simulink model "water_hopper_cpg"  (Simulink 8.0)
settings: Solver=ode23t  StartTime=0.0  StopTime=5  MaxStep=1e-3  RelTol=1e-9
values from neighbouring files (symbols this model uses):
  alpha = 30    [SimParam.m]    (also in SimParam_cpg.m)
  Amp = coeff(1)    [SSheight3.m]    (also in SimParam.m = 0.0249; SimParam_cpg.m = 0.0249; TwoD_search.m = AMP(jj,1); linear_search.m = leg_length/4)
  amp = Amp    (= 0.0249)    [SimParam.m]    (also in SimParam_cpg.m)
  b = 0.5*C_d*S*density    [SSheight.m]    (also in SSheight12.m; SSheight2.m; SSheight3.m; SSpower.m)
  C_d = 0.703    [SSheight.m]    (also in SSheight12.m; SSheight2.m; SSheight3.m; SSpower.m)
  density = 1000    [SSheight.m]    (also in SSheight12.m; SSheight2.m; SSheight3.m; SSpower.m)
  Fratio = (r2^2)/(r1^2)    (= 0.0625)    [SimParam_cpg.m]
  freq = 84    [SimParam_cpg.m]    (also in TwoD_search.m = FREQ(1,kk); height_search.m = FREQ(k); height_search2.m = freqs(k); linear_search.m = FREQ(2:end))
  g = 9.81    [SSheight.m]    (also in SSheight12.m; SSheight2.m; SSheight3.m; SSpower.m)
  k = C_d*S*density*g    [SSheight.m]    (also in SSheight12.m; SSheight2.m; SSheight3.m; SSpower.m)
  leg_length = Amp    (= 0.0249)    [SimParam.m]    (also in SimParam_2G.m = 0.1; SimParam_cpg.m; height_search.m = Amp)
  mass = 0.025    [SimParam.m]    (also in SimParam_cpg.m)
  omega_0 = [65 65]'    [SimParam_cpg.m]
  S1 = (pi*r1^2)*area    (= 0.00115422114093)    [SimParam.m]    (also in SimParam_cpg.m)
  S2 = (pi*r2^2)*area    (= 7.21388213081e-05)    [SimParam.m]    (also in SimParam_cpg.m)
  tau = 0.001    [SimParam.m]    (also in SimParam_cpg.m)
  y_0 = Amp/2    (= 0.01245)    [SimParam.m]    (also in SimParam_2G.m = 0.1; SimParam_cpg.m; height_search.m = Amp/2; height_search2.m = Amp/2)
libraries: mblibv1 x13, simulink x2, dspinverses x1, powerlib_extras x1
settings Model: Creator=Metti  LastModifiedBy=nitisht
settings SolverCC: ZeroCrossControl=DisableAll
settings DataIOCC: SignalLoggingSaveFormat=ModelDataLogs
settings DebuggingCC: FcnCallInpInsideContextMsg=EnableAllAsWarning
settings SimMechanicsCC: VisSampleTime=0.05  AutoFitVis=GROWTOFIT  LastVizWinPosition=[520 378 560 420]  CamPosition=[0;32.5432;11.11;]  CamTarget=[0;32.5432;0;]  CamUpVector=[0;1;0;]  CamHeight=0.102  VisBackgroundColor=[0.9;0.9;0.95;]  DefaultBodyColor=[1;0;0;]
settings ConfigurationSet: Description=SimMechanics 2G

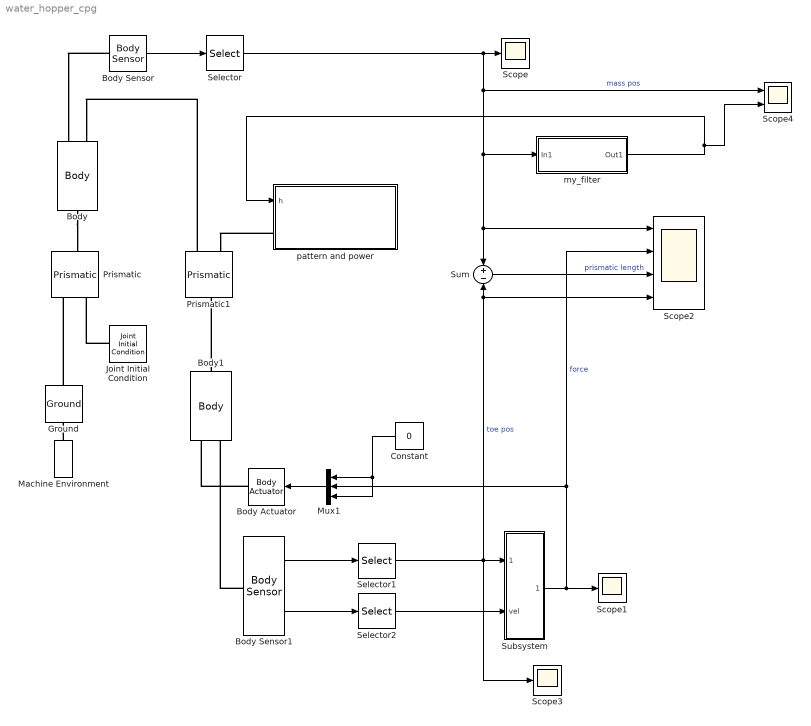
== system water_hopper_cpg ==
  Body : mblibv1/Bodies/Body  LConnTagsString=CS1  RConnTagsString=CS2|CS3  UpdateFromCAD=off  DialogClass=MechanicalBodyBlock  Mass=mass  MassUnits=kg  InertiaUnits=kg*m^2  Inertia=eye(3)  Shape=Cylinder  ShapeDims=[1 1]  ShapeUnits=m  ShapeUse=false  Density=1  DensityUnits=kg/m^3  DensityUse=false  GraphicsMode=MACHINE_DEFAULT  BodyColorSelMode=MACHINE_DEFAULT  BodyColor=[1 0 0]  AttachedToCS=CG  CG=Left$CG$[0 0 0]$WORLD$WORLD$m$[0 0 0]$Euler X-Y-Z$deg$WORLD$false$none  WorkingFrames=Left$CS1$[0 0 0]$CG$CG$m$[0 0 0]$Euler X-Y-Z$deg$WORLD$true$none#Right$CS2$[0 0 0]$CG$CG$m$[0 0 0]$Euler X-Y-Z$deg$WORLD$true$none#Right$CS3$[0 0 0]$CG$CG$m$[0 0 0]$Euler X-Y-Z$deg$WORLD$true$none  CGPos=[0 0 0]  CGRot=[0 0 0]  CS0Pos=[]  CS0Rot=[]  CS1Pos=[0 0 0]  CS1Rot=[0 0 0]  CS2Pos=[0 0 0]  CS2Rot=[0 0 0]  CS3Pos=[0 0 0]  CS3Rot=[0 0 0]  CS4Pos=[]  CS4Rot=[]  CS5Pos=[]  CS5Rot=[]  CS6Pos=[]  CS6Rot=[]  CS7Pos=[]  CS7Rot=[]  CS8Pos=[]  CS8Rot=[]  CS9Pos=[]  CS9Rot=[]  CS10Pos=[]  CS10Rot=[]  CS11Pos=[]  CS11Rot=[]  CS12Pos=[]  CS12Rot=[]  CS13Pos=[]  CS13Rot=[]  CS14Pos=[]  CS14Rot=[]  CS15Pos=[]  CS15Rot=[]  CS16Pos=[]  CS16Rot=[]  CS17Pos=[]  CS17Rot=[]  CS18Pos=[]  CS18Rot=[]  CS19Pos=[]  CS19Rot=[]  CS20Pos=[]  CS20Rot=[]
  Body Actuator : mblibv1/Sensors &  Actuators/Body Actuator  UpdateFromCAD=off  PhysicalDomain=Mechanical  PortType=blob  ActuationStyle=Force  AngleUnits=deg  ArcVelocityUnits=deg/s  ArcAccelerationUnits=deg/s^2  CoordPositionUnits=m  VelocityUnits=m/s  AccelerationUnits=m/s^2  ForceUnits=N  TorqueUnits=N-m  ActiveIO=on  Width=3  DialogClass=MechanicalActuatorBlock  ReferenceFrame=Absolute (World)  Angle=off  CoordPosition=on  Force=on  Torque=off
  Body Sensor : mblibv1/Sensors &  Actuators/Body Sensor  UpdateFromCAD=off  PhysicalDomain=Mechanical  PortType=blob  Muxed=on  Pose=off  Angle=on  AngleUnits=deg  ArcVelocity=off  ArcVelocityUnits=deg/s  ArcAcceleration=off  ArcAccelerationUnits=deg/s^2  CoordPosition=on  CoordPositionUnits=m  Velocity=off  VelocityUnits=m/s  Acceleration=off  AccelerationUnits=m/s^2  Quaternion=on  QuaternionDT=off  QuaternionDDT=off  QuaternionUnits=off  OutputVector=[1]  ActiveIO=on  Width=3  DialogClass=MechanicalSensorBlock  ReferenceFrame=Absolute (World)
  Body Sensor1 : mblibv1/Sensors &  Actuators/Body Sensor  UpdateFromCAD=off  PhysicalDomain=Mechanical  PortType=blob  Muxed=off  Pose=off  Angle=on  AngleUnits=deg  ArcVelocity=off  ArcVelocityUnits=deg/s  ArcAcceleration=off  ArcAccelerationUnits=deg/s^2  CoordPosition=on  CoordPositionUnits=m  Velocity=on  VelocityUnits=m/s  Acceleration=off  AccelerationUnits=m/s^2  Quaternion=on  QuaternionDT=off  QuaternionDDT=off  QuaternionUnits=off  OutputVector=[1]  ActiveIO=on  Width=6  DialogClass=MechanicalSensorBlock  ReferenceFrame=Absolute (World)
  Body1 : mblibv1/Bodies/Body  LConnTagsString=CS1  RConnTagsString=CS2|CS3  UpdateFromCAD=off  DialogClass=MechanicalBodyBlock  Mass=0  MassUnits=kg  InertiaUnits=kg*m^2  Inertia=eye(3)  Shape=Cylinder  ShapeDims=[1 1]  ShapeUnits=m  ShapeUse=false  Density=1  DensityUnits=kg/m^3  DensityUse=false  GraphicsMode=MACHINE_DEFAULT  BodyColorSelMode=MACHINE_DEFAULT  BodyColor=[1 0 0]  AttachedToCS=CG  CG=Left$CG$[0 -leg_length 0]$CS1$CS1$m$[0 0 0]$Euler X-Y-Z$deg$WORLD$false$none  WorkingFrames=Left$CS1$[0 0 0]$Adjoining$Adjoining$m$[0 0 0]$Euler X-Y-Z$deg$WORLD$true$none#Right$CS2$[0 -leg_length 0]$CS1$CS1$m$[0 0 0]$Euler X-Y-Z$deg$WORLD$true$none#Right$CS3$[0 -leg_length 0]$CS1$CS1$m$[0 0 0]$Euler X-Y-Z$deg$WORLD$true$none  CGPos=[0 -leg_length 0]  CGRot=[0 0 0]  CS0Pos=[]  CS0Rot=[]  CS1Pos=[0 0 0]  CS1Rot=[0 0 0]  CS2Pos=[0 -leg_length 0]  CS2Rot=[0 0 0]  CS3Pos=[0 -leg_length 0]  CS3Rot=[0 0 0]  CS4Pos=[]  CS4Rot=[]  CS5Pos=[]  CS5Rot=[]  CS6Pos=[]  CS6Rot=[]  CS7Pos=[]  CS7Rot=[]  CS8Pos=[]  CS8Rot=[]  CS9Pos=[]  CS9Rot=[]  CS10Pos=[]  CS10Rot=[]  CS11Pos=[]  CS11Rot=[]  CS12Pos=[]  CS12Rot=[]  CS13Pos=[]  CS13Rot=[]  CS14Pos=[]  CS14Rot=[]  CS15Pos=[]  CS15Rot=[]  CS16Pos=[]  CS16Rot=[]  CS17Pos=[]  CS17Rot=[]  CS18Pos=[]  CS18Rot=[]  CS19Pos=[]  CS19Rot=[]  CS20Pos=[]  CS20Rot=[]
  Constant : Constant  Value=0
  Ground : mblibv1/Bodies/Ground  UpdateFromCAD=off  LeftPortType=env  RightPortType=workingframe  PhysicalDomain=Mechanical  DialogClass=GroundBlock  CoordPosition=[0 0 0]  CoordPositionUnits=m  StateVectorMgrId=1  MachineId=[2 0]  ShowEnvPort=on
  Joint Initial Condition : mblibv1/Sensors &  Actuators/Joint Initial Condition  UpdateFromCAD=off  LeftPortType=blob  RightPortType=blob  PhysicalDomain=mechanical  DialogClass=InitialConditionBlock  InitialConditions=P1$true$y_0$m$deg$0$m/s$deg/s#P2$false$0$m$deg$0$m/s$deg/s#P3$false$0$m$deg$0$m/s$deg/s#R1$false$0$m$deg$0$m/s$deg/s#R2$false$0$m$deg$0$m/s$deg/s#R3$false$0$m$deg$0$m/s$deg/s#S$false$0$m$deg$0$m/s$deg/s  P1PIC=y_0  P1VIC=0  P2PIC=0  P2VIC=0  P3PIC=0  P3VIC=0  R1PIC=0  R1VIC=0  R2PIC=0  R2VIC=0  R3PIC=0  R3VIC=0  SPIC=0  SVIC=0
  Machine Environment : mblibv1/Bodies/Machine Environment  PortType=env  PhysicalDomain=Mechanical  DialogTemplateClass=MECH.MachineEnvironment  SyncWhenCopied=off  Gravity=[0 -g 0]  GravityUnits=m/s^2  GravityAsSignal=off  Dimensionality=Auto-detect  AnalysisType=Forward dynamics  LinearAssemblyTolerance=1e-3  LinearAssemblyToleranceUnits=m  AngularAssemblyTolerance=1e-3  AngularAssemblyToleranceUnits=rad  ConstraintSolverType=Stabilizing  ConstraintRelTolerance=1e-4  ConstraintAbsTolerance=1e-4  UseRobustSingularityHandling=off  RedundancyAnalysisToleranceType=Automatically select tolerance  RedundancyAnalysisTolerance=1e-14  StatePerturbationType=Fixed  PerturbationSize=1e-5  VisualizeMachine=on  BodyVisualizationType=Use model default body geometries  BodyColorSelMode=Use model default  DefaultBodyColor=[1 0 0]
  Mux1 : Mux  Inputs=3
  Prismatic : mblibv1/Joints/Prismatic  LConnTagsString=__newl0|SA1  RConnTagsString=__newr0  UpdateFromCAD=off  NumSAPorts=1  CutJoint=off  MarkAsCut=off  Primitives=prismatic  PrimitiveProps=P1$World$[0 1 0]$prismatic  DialogClass=JointBlock  P1Axis=[0 1 0]
  Prismatic1 : mblibv1/Joints/Prismatic  LConnTagsString=__newl0|SA1  RConnTagsString=__newr0  UpdateFromCAD=off  NumSAPorts=1  CutJoint=off  MarkAsCut=off  Primitives=prismatic  PrimitiveProps=P1$World$[0 1 0]$prismatic  DialogClass=JointBlock  P1Axis=[0 1 0]
  Scope : Scope
      settings: YMin=-0.053045  YMax=-0.053005  SaveName=ball_position
  Scope1 : Scope
      settings: SaveName=force
  Scope2 : Scope  NumInputPorts=4
      settings: YMin=-5~-5~-5~-5  YMax=5~5~5~5  SaveName=ScopeData2
  Scope3 : Scope
      settings: SaveName=toe_position
  Scope4 : Scope  NumInputPorts=2
      settings: YMin=-0.015~0.009  YMax=0.03~0.02  SaveName=ball_position1
  Selector : Selector  InputPortWidth=3  IndexOptions=Index vector (dialog)  Indices=[2]  OutputSizes=1
  Selector1 : Selector  InputPortWidth=3  IndexOptions=Index vector (dialog)  Indices=[2]  OutputSizes=1
  Selector2 : Selector  InputPortWidth=3  IndexOptions=Index vector (dialog)  Indices=[2]  OutputSizes=1
  Subsystem : Subsystem
  Sum : Sum  Inputs=+|-
  my_filter : Subsystem
  pattern and power : Subsystem
  wires:
  Body Sensor/1 -> Selector/1
  Selector/1 -> Scope/1, Scope4/1, Scope2/1, Sum/1, my_filter/1(In1)  "mass pos"
  Body Sensor1/1 -> Selector1/1
  Body Sensor1/2 -> Selector2/1
  Selector1/1 -> Sum/2, Scope2/4, Subsystem/1(pos), Scope3/1  "toe pos"
  Selector2/1 -> Subsystem/2(vel)
  Subsystem/1(force) -> Scope1/1, Mux1/2, Scope2/2  "force"
  Mux1/1 -> Body Actuator/1
  Constant/1 -> Mux1/1, Mux1/3
  Sum/1 -> Scope2/3  "prismatic length"
  my_filter/1(Out1) -> pattern and power/1(h), Scope4/2
  connections:
  Body Sensor/LConn1 -- Body/RConn1
  Body/LConn1 -- Prismatic/RConn1
  Machine Environment/RConn1 -- Ground/LConn1
  Ground/RConn1 -- Prismatic/LConn1
  Body1/LConn1 -- Prismatic1/RConn1
  Body Actuator/RConn1 -- Body1/RConn1
  Body Sensor1/LConn1 -- Body1/RConn2
  Prismatic1/LConn1 -- Body/RConn2
  Joint Initial Condition/RConn1 -- Prismatic/LConn2
  pattern and power/LConn1 -- Prismatic1/LConn2

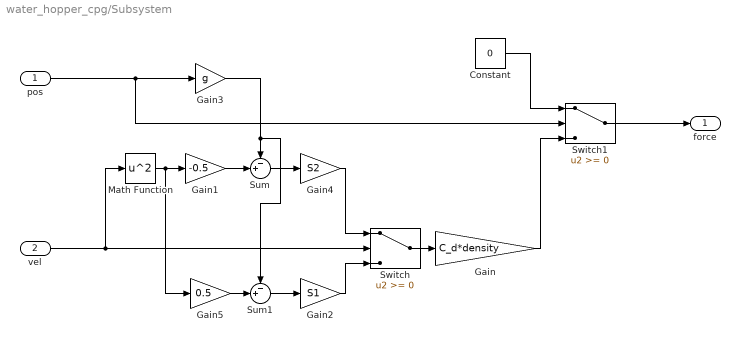
== system water_hopper_cpg/Subsystem ==
  pos : Inport
  vel : Inport  Port=2
  Constant : Constant  Value=0
  Gain : Gain  Gain=C_d*density
  Gain1 : Gain  Gain=-0.5
  Gain2 : Gain  Gain=S1
  Gain3 : Gain  Gain=g
  Gain4 : Gain  Gain=S2
  Gain5 : Gain  Gain=0.5
  Math Function : Math  Operator=square  SaturateOnIntegerOverflow=on
  Sum : Sum  Inputs=-+|
  Sum1 : Sum  Inputs=-+|
  Switch : Switch  ZeroCross=off
  Switch1 : Switch
  force : Outport
  wires:
  vel/1 -> Switch/2, Math Function/1
  Math Function/1 -> Gain1/1, Gain5/1
  Gain1/1 -> Sum/2
  pos/1 -> Gain3/1, Switch1/2
  Gain3/1 -> Sum/1, Sum1/1
  Sum/1 -> Gain4/1
  Gain4/1 -> Switch/1
  Gain2/1 -> Switch/3
  Switch/1 -> Gain/1
  Switch1/1 -> force/1
  Gain/1 -> Switch1/3
  Constant/1 -> Switch1/1
  Sum1/1 -> Gain2/1
  Gain5/1 -> Sum1/2

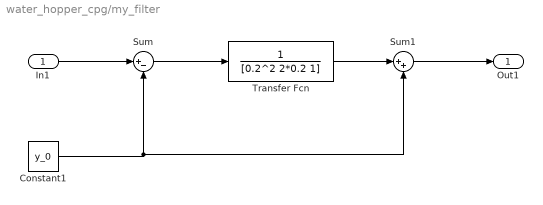
== system water_hopper_cpg/my_filter ==
  In1 : Inport
  Constant1 : Constant  Value=y_0
  Sum : Sum  Inputs=|+-
  Sum1 : Sum  Inputs=|++
  Transfer Fcn : TransferFcn  Denominator=[0.2^2 2*0.2 1]
  Out1 : Outport
  wires:
  Constant1/1 -> Sum1/2, Sum/2
  In1/1 -> Sum/1
  Sum/1 -> Transfer Fcn/1
  Transfer Fcn/1 -> Sum1/1
  Sum1/1 -> Out1/1

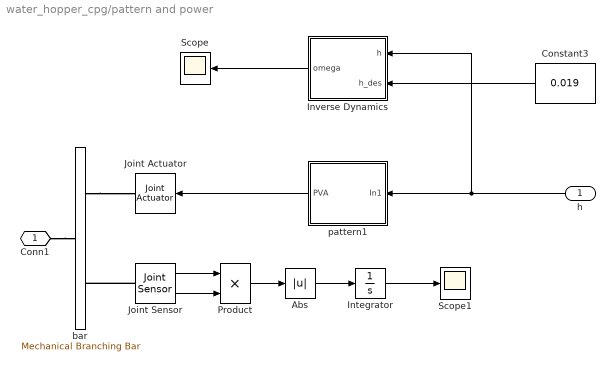
== system water_hopper_cpg/pattern and power ==
  h : Inport
  Abs : Abs
  Constant3 : Constant  Value=0.019
  Integrator : Integrator
  Inverse Dynamics : Subsystem
  Joint Actuator : mblibv1/Sensors &  Actuators/Joint Actuator  UpdateFromCAD=off  PhysicalDomain=Mechanical  PortType=blob  ActuationStyle=Motion  AngleUnits=deg  ArcVelocityUnits=deg/s  ArcAccelerationUnits=deg/s^2  CoordPositionUnits=m  VelocityUnits=m/s  AccelerationUnits=m/s^2  ForceUnits=N  TorqueUnits=N*m  ActiveIO=on  Width=3  DialogClass=MechanicalActuatorBlock  Primitive=P1  ReferenceFrame=Absolute (World)
  Joint Sensor : mblibv1/Sensors &  Actuators/Joint Sensor  UpdateFromCAD=off  PhysicalDomain=Mechanical  PortType=blob  Muxed=off  Pose=off  Angle=on  AngleUnits=deg  ArcVelocity=off  ArcVelocityUnits=deg/s  ArcAcceleration=off  ArcAccelerationUnits=deg/s^2  CoordPosition=off  CoordPositionUnits=m  Velocity=on  VelocityUnits=m/s  Acceleration=off  AccelerationUnits=m/s^2  Quaternion=on  QuaternionDT=off  QuaternionDDT=off  QuaternionUnits=off  OutputVector=[1]  ActiveIO=on  Width=2  DialogClass=MechanicalSensorBlock  Primitive=P1  Force=on  ForceUnits=N  Torque=off  TorqueUnits=N*m  ReferenceFrame=Absolute (World)  ReactionSensedSide=Base  ReactionReferenceFrame=Absolute (World)  ReactionForce=off  ReactionForceUnits=N  ReactionMoment=off  ReactionMomentUnits=N*m
  Product : Product  RndMeth=Zero
  Scope : Scope
      settings: YMin=62.5  YMax=90  SaveName=ScopeData5
  Scope1 : Scope
      settings: SaveName=Work
  bar : mblibv1/Utilities/Mechanical Branching Bar  LConnTagsString=_newl0  RConnTagsString=SA0|SA1  UpdateFromCAD=off  DialogClass=MechanicalBranchingBarBlock  NumSAPorts=2
  pattern1 : Subsystem  mask{Amp=amp, Offset=0, freq=freq}
      mask prompts: Amp "Amplitude"; freq "Frequency"
      mask TypeOptions freq: Constant/Value
  Conn1 : PMIOPort  Port=1  Side=Left
  wires:
  pattern1/1(PVA) -> Joint Actuator/1
  Joint Sensor/1 -> Product/1
  Product/1 -> Abs/1
  Abs/1 -> Integrator/1
  Integrator/1 -> Scope1/1
  Joint Sensor/2 -> Product/2
  h/1 -> Inverse Dynamics/1(h), pattern1/1(In1)
  Constant3/1 -> Inverse Dynamics/2(h_des)
  Inverse Dynamics/1(omega) -> Scope/1
  connections:
  bar/RConn1 -- Joint Actuator/RConn1
  Joint Sensor/LConn1 -- bar/RConn2
  Conn1/RConn1 -- bar/LConn1

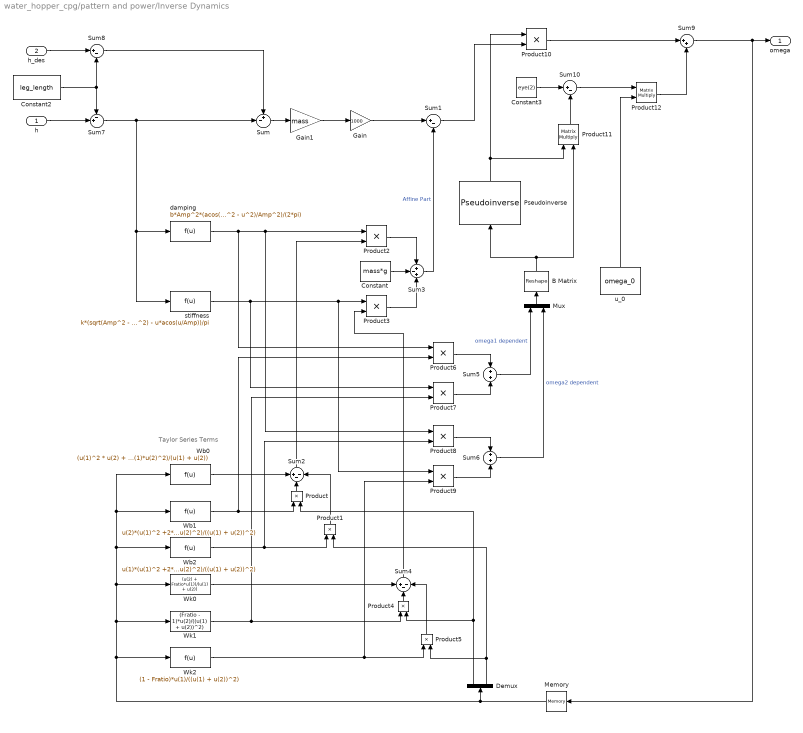
== system water_hopper_cpg/pattern and power/Inverse Dynamics ==
  note: Taylor Series Terms
  h : Inport
  h_des : Inport  Port=2
  B Matrix : Reshape  OutputDimensionality=Customize  OutputDimensions=[1,2]
  Constant : Constant  Value=mass*g
  Constant2 : Constant  Value=leg_length
  Constant3 : Constant  Value=eye(2)
  Demux : Demux  Outputs=2
  Gain : Gain  Gain=1000
  "Gain1 " : Gain  Gain=mass
  Memory : Memory  X0=omega_0
  Mux : Mux  Inputs=2
  Product{,1..10} (11 alike) : Product  RndMeth=Zero
  Product11 : Product  Multiplication=Matrix(*)  RndMeth=Zero
  Product12 : Product  Multiplication=Matrix(*)  RndMeth=Zero
  Pseudoinverse : dspinverses/Pseudoinverse  wanterr=off
  Sum : Sum  Inputs=+-|
  Sum1 : Sum  Inputs=|+-
  Sum10 : Sum  Inputs=|+-
  Sum2 : Sum  Inputs=+--
  Sum3 : Sum  Inputs=+-+
  Sum4 : Sum  Inputs=+--
  Sum5 : Sum  Inputs=+|+
  Sum6 : Sum  Inputs=+|+
  Sum7 : Sum  Inputs=-+|
  Sum8 : Sum  Inputs=|+-
  Sum9 : Sum  Inputs=|++
  Wb0 : Fcn  Expr=(u(1)^2 * u(2) + Fratio*u(1)*u(2)^2)/(u(1) + u(2))
  Wb1 : Fcn  Expr=u(2)*(u(1)^2 +2*u(1)*u(2) + Fratio*u(2)^2)/((u(1) + u(2))^2)
  Wb2 : Fcn  Expr=u(1)*(u(1)^2 +2*Fratio*u(1)*u(2) + Fratio*u(2)^2)/((u(1) + u(2))^2)
  Wk0 : Fcn  Expr=(u(2) + Fratio*u(1))/(u(1) + u(2))
  Wk1 : Fcn  Expr=(Fratio - 1)*u(2)/((u(1) + u(2))^2)
  Wk2 : Fcn  Expr=(1 - Fratio)*u(1)/((u(1) + u(2))^2)
  damping : Fcn  Expr=b*Amp^2*(acos(u/Amp) - u*sqrt(Amp^2 - u^2)/Amp^2)/(2*pi)
  stiffness : Fcn  Expr=k*(sqrt(Amp^2 - u^2) - u*acos(u/Amp))/pi
  u_0 : Constant  Value=omega_0  VectorParams1D=off
  omega : Outport
  wires:
  Memory/1 -> Wb0/1, Wb1/1, Wb2/1, Wk0/1, Wk1/1, Wk2/1, Demux/1
  "Gain1 "/1 -> Gain/1
  Gain/1 -> Sum1/1
  Sum/1 -> "Gain1 "/1
  Wb0/1 -> Sum2/1
  Product/1 -> Sum2/2
  Wb1/1 -> Product6/2, Product/1
  Demux/1 -> Product/2, Product4/2
  Wb2/1 -> Product8/2, Product1/1
  Product1/1 -> Sum2/3
  Demux/2 -> Product5/2, Product1/2
  damping/1 -> Product6/1, Product8/1, Product2/1
  Sum2/1 -> Product2/2
  stiffness/1 -> Product7/1, Product9/1, Product3/1
  Wk0/1 -> Sum4/1
  Wk1/1 -> Product7/2, Product4/1
  Wk2/1 -> Product9/2, Product5/1
  Product4/1 -> Sum4/2
  Product5/1 -> Sum4/3
  Sum4/1 -> Product3/2
  Product2/1 -> Sum3/1
  Sum3/1 -> Sum1/2  "Affine Part"
  Product3/1 -> Sum3/3
  Constant/1 -> Sum3/2
  Product6/1 -> Sum5/1
  Product7/1 -> Sum5/2
  Product9/1 -> Sum6/2
  Product8/1 -> Sum6/1
  Sum5/1 -> Mux/1  "omega1 dependent"
  Sum6/1 -> Mux/2  "omega2 dependent"
  Mux/1 -> B Matrix/1
  B Matrix/1 -> Product11/2, Pseudoinverse/1
  Sum7/1 -> Sum/2, damping/1, stiffness/1
  h/1 -> Sum7/2
  Constant2/1 -> Sum8/2, Sum7/1
  h_des/1 -> Sum8/1
  Sum8/1 -> Sum/1
  Pseudoinverse/1 -> Product11/1, Product10/1
  Sum1/1 -> Product10/2
  Product10/1 -> Sum9/1
  Product11/1 -> Sum10/2
  Constant3/1 -> Sum10/1
  Sum10/1 -> Product12/1
  u_0/1 -> Product12/2
  Product12/1 -> Sum9/2
  Sum9/1 -> Memory/1, omega/1

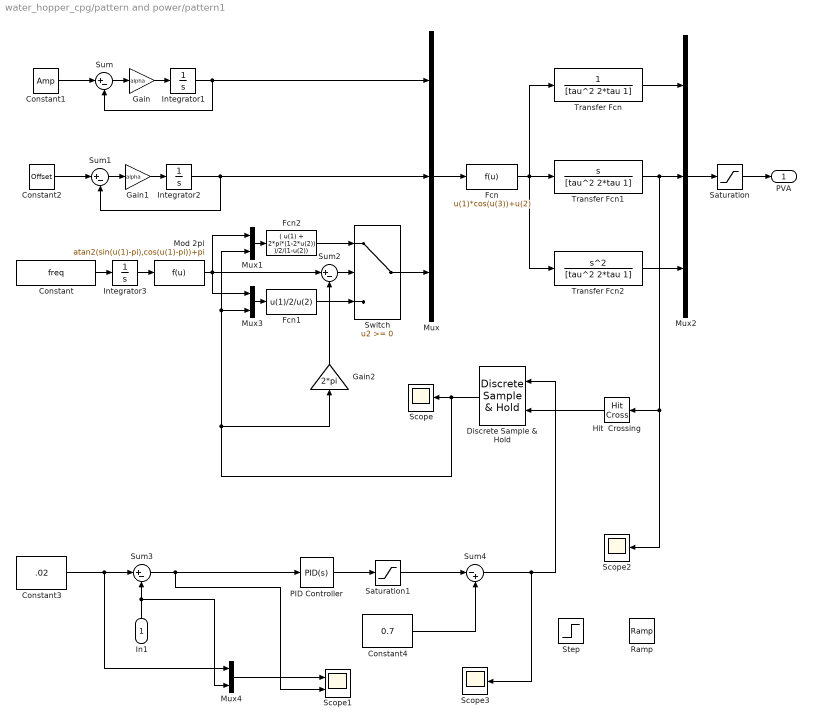
== system water_hopper_cpg/pattern and power/pattern1 ==
  In1 : Inport
  Constant : Constant  Value=freq
  Constant1 : Constant  Value=Amp
  Constant2 : Constant  Value=Offset
  Constant3 : Constant  Value=.02
  Constant4 : Constant  Value=0.7
  Discrete Sample & Hold : powerlib_extras/Discrete  Control Blocks/Discrete Sample & Hold  ic=0  Ts=50e-6
  Fcn : Fcn  Expr=u(1)*cos(u(3))+u(2)
  Fcn1 : Fcn  Expr=u(1)/2/u(2)
  Fcn2 : Fcn  Expr=( u(1) + 2*pi*(1-2*u(2)) )/2/(1-u(2))
  Gain : Gain  Gain=alpha
  Gain1 : Gain  Gain=alpha
  Gain2 : Gain  Gain=2*pi
  Hit  Crossing : HitCross  HitCrossingDirection=falling
  Integrator1 : Integrator
  Integrator2 : Integrator
  Integrator3 : Integrator  InitialCondition=0.01*rand
  Mod 2pi : Fcn  Expr=atan2(sin(u(1)-pi),cos(u(1)-pi))+pi
  Mux : Mux  Inputs=3
  Mux1 : Mux  Inputs=2
  Mux2 : Mux  Inputs=3
  Mux3 : Mux  Inputs=2
  Mux4 : Mux  Inputs=2
  PID Controller : simulink/Continuous/PID Controller  Controller=PID  TimeDomain=Continuous-time  SampleTime=1  IntegratorMethod=Forward Euler  FilterMethod=Forward Euler  Form=Parallel  P=5  I=0.1  D=0.5  N=100  InitialConditionSource=internal  InitialConditionForIntegrator=0  InitialConditionForFilter=0  ExternalReset=none  LimitOutput=off  UpperSaturationLimit=inf  LowerSaturationLimit=-inf  LinearizeAsGain=on  AntiWindupMode=none  Kb=1  TrackingMode=off  Kt=1  PParamMin=[]  PParamMax=[]  IParamMin=[]  IParamMax=[]  DParamMin=[]  DParamMax=[]  NParamMin=[]  NParamMax=[]  KbParamMin=[]  KbParamMax=[]  KtParamMin=[]  KtParamMax=[]  POutMin=[]  POutMax=[]  IOutMin=[]  IOutMax=[]  DOutMin=[]  DOutMax=[]  NOutMin=[]  NOutMax=[]  KbOutMin=[]  KbOutMax=[]  KtOutMin=[]  KtOutMax=[]  IntegratorOutMin=[]  IntegratorOutMax=[]  FilterOutMin=[]  FilterOutMax=[]  SumOutMin=[]  SumOutMax=[]  SumI1OutMin=[]  SumI1OutMax=[]  SumI2OutMin=[]  SumI2OutMax=[]  SumI3OutMin=[]  SumI3OutMax=[]  SumDOutMin=[]  SumDOutMax=[]  SaturationOutMin=[]  SaturationOutMax=[]  IntegratorContinuousStateAttributes=''  IntegratorStateMustResolveToSignalObject=off  IntegratorRTWStateStorageClass=Auto  FilterContinuousStateAttributes=''  FilterStateMustResolveToSignalObject=off  FilterRTWStateStorageClass=Auto
  Ramp : simulink/Sources/Ramp  slope=0.4/20  start=0  X0=0.3
  Saturation : Saturate  UpperLimit=3*amp*freq^2  LowerLimit=-3*amp*freq^2
  Saturation1 : Saturate  UpperLimit=0.3  LowerLimit=-0.3
  Scope : Scope
  Scope1 : Scope  NumInputPorts=2
      settings: YMin=-5~-5  YMax=5~5
  Scope2 : Scope
      settings: SaveName=ScopeData3
  Scope3 : Scope
      settings: SaveName=ScopeData4
  Step : Step  Time=2  Before=0.4  After=0.6  SampleTime=0
  Sum{,1..3} (4 alike) : Sum  Inputs=|+-
  Sum4 : Sum  Inputs=|-+
  Switch : Switch
  Transfer Fcn : TransferFcn  Denominator=[tau^2 2*tau 1]
  Transfer Fcn1 : TransferFcn  Numerator=[1 0]  Denominator=[tau^2 2*tau 1]
  Transfer Fcn2 : TransferFcn  Numerator=[1 0 0]  Denominator=[tau^2 2*tau 1]
  PVA : Outport
  wires:
  Constant/1 -> Integrator3/1
  Mod 2pi/1 -> Mux1/1, Mux3/1, Sum2/1
  Integrator3/1 -> Mod 2pi/1
  Switch/1 -> Mux/3
  Fcn1/1 -> Switch/3
  Fcn2/1 -> Switch/1
  Mux/1 -> Fcn/1
  Gain1/1 -> Integrator2/1
  Constant2/1 -> Sum1/1
  Integrator2/1 -> Mux/2, Sum1/2
  Sum1/1 -> Gain1/1
  Gain/1 -> Integrator1/1
  Constant1/1 -> Sum/1
  Integrator1/1 -> Mux/1, Sum/2
  Sum/1 -> Gain/1
  Transfer Fcn2/1 -> Mux2/3
  Transfer Fcn/1 -> Mux2/1
  Transfer Fcn1/1 -> Scope2/1, Hit  Crossing/1, Mux2/2
  Mux2/1 -> Saturation/1
  Fcn/1 -> Transfer Fcn1/1, Transfer Fcn/1, Transfer Fcn2/1
  Saturation/1 -> PVA/1
  Hit  Crossing/1 -> Discrete Sample & Hold/2
  Sum2/1 -> Switch/2
  Gain2/1 -> Sum2/2
  Discrete Sample & Hold/1 -> Mux3/2, Mux1/2, Gain2/1, Scope/1
  Mux1/1 -> Fcn2/1
  Mux3/1 -> Fcn1/1
  In1/1 -> Mux4/2, Sum3/2
  Constant3/1 -> Mux4/1, Sum3/1
  Sum3/1 -> Scope1/2, PID Controller/1
  Saturation1/1 -> Sum4/1
  PID Controller/1 -> Saturation1/1
  Mux4/1 -> Scope1/1
  Constant4/1 -> Sum4/2
  Sum4/1 -> Scope3/1, Discrete Sample & Hold/1
